simulink model "DesignTemperatureControlForDataCenter"  (R2025b)
settings: Solver=daessc  StartTime=0.0  StopTime=3600*4  FixedStep=0.5  MaxStep=1  RelTol=1e-3  AbsTol=1e-3
PreLoadFcn:
  | if ~exist("modelParam")
  |     setDefaultParameters;
  | end
undefined symbols (not defined in the file or in its folder): DiscIntNeverNeededParam, modelParam, value
libraries: fl_lib x78, nesl_utility x18, SimscapeFluids_lib x11, datacenter_lib x9, simulink_extras x4, slpidlib x2
(part 1 of 3)
settings Model: Creator=vikrants  LastModifiedBy=vikrants
settings SolverCC: AutoScaleAbsTol=off  NumberNewtonIterations=5.0  MaxConsecutiveMinStep=10  AlgebraicLoopSolver=TrustRegion  MaxZcPerStep=1.0
settings DataIOCC: SaveOutput=off  DSMLogging=off  SaveTime=off  ReturnWorkspaceOutputs=off  SignalLoggingName=logsout_DesignTemperatureControllerDataCenter
settings DebuggingCC: UnconnectedInputMsg=warning  UnconnectedOutputMsg=warning  UnconnectedLineMsg=warning  SymbolicDimsDataTypeCodeGenerationDiagnostic=none
settings ModelReferenceCC: EnableRefExpFcnMdlSchedulingChecks=on
settings SFSimCC: CustomCodeUndefinedFunction=UseInterfaceOnly
settings RTWCC: GPUComputeCapability=3.5  DLArmComputeVersion=19.05
settings SimscapeCC: SimscapeLogLimitData=off  SimscapeLogDataHistory=10000.0

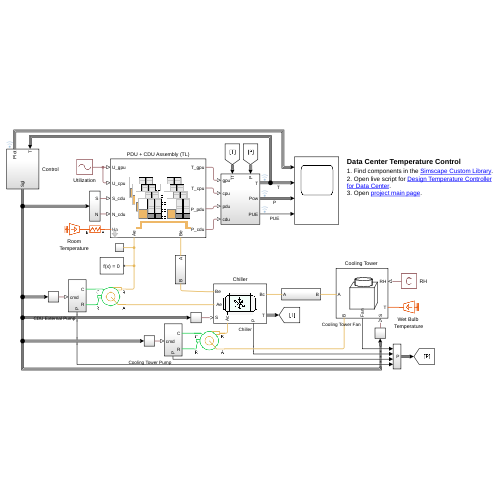
[thumbnail: Simulink's stored preview of the top-level diagram]
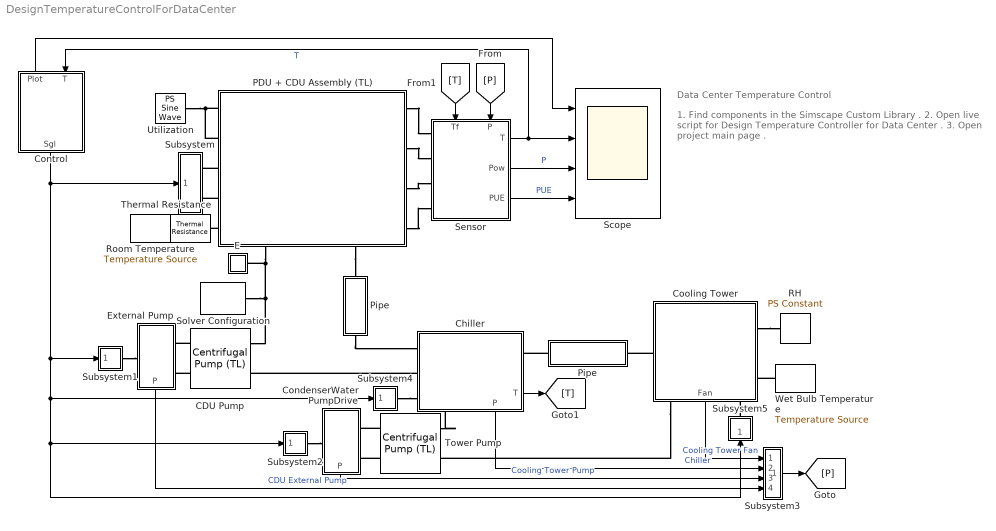
== system DesignTemperatureControlForDataCenter ==
  note: Data Center Temperature Control
  note: 1. Find components in the Simscape Custom Library .
      | 2. Open live script for Design Temperature Controller for Data Center .
      | 3. Open project main page .
  CDU Pump : SimscapeFluids_lib/Thermal Liquid/Pumps & Motors/Centrifugal Pump (TL)  pump_parameterization=fluids.thermal_liquid.pumps_motors.enum.CentrifugalPumpParameterization.Nominal  capacity_ref_nominal=5736% 07-Oct-2026 22:51:40 lpm  head_ref_nominal=33 m  power_ref_nominal=100 kW  head_ref_max=48 m  capacity_ref_max=16520% 07-Oct-2026 22:51:40 lpm  omega_ref_analytic=2400 rpm  flow_rate_1D_TLU=[16.67, 30, 40, 53.33, 66.67, 83.33] lpm  head_1D_TLU=[50, 47.5, 45, 40, 35, 25] m  power_1D_TLU=[.6, .75, .85, .93, .98, .99] kW  omega_ref_1D=3500 rpm  rho_ref_1D=998.21 kg/m^3  omega_threshold_factor=1e-2  flow_rate_2D_TLU=[16.67, 23.33, 30, 40, 53.33, 60] lpm  omega_2D_TLU=[2450, 2800, 3150, 3500] rpm  head_2D_TLU=[25, 32.7, 42.5, 50; 24, 31.7, 41, 49; 22.7, 30.5, 39, 47.5; 20, 28, 36, 45; 15.7, 24, 32, 40; 12.5, 21, 29.5, 37.5] m  power_2D_TLU=[.28, .38, .5, .6; .31, .41, .55, .68; .33, .44, .6, .75; .36, .48, .65, .83; .38, .53, .72, .93; .39, .55, .75, .97] kW  rho_ref_2D=998.21 kg/m^3  diameter_ratio=1  mech_orientation=fluids.thermal_liquid.pumps_motors.enum.CentrifugalPumpMechOrientation.Positive  area=0.01 m^2  operation_check=simscape.enum.assert.action.none
      settings: InternalSimscapePortConfiguration="{\"Bottom\":[],\"Left\":[{\"id\":\"A\",\"label\":\"A\",\"type\":\"foundation.thermal_liquid.thermal_liquid\"},{\"id\":\"B\",\"label\":\"B\",\"type\":\"foundation.thermal_liquid.thermal_liquid\"}],\"Right\":[{\"id\":\"R\",\"label\":\"R\",\"type\":\"foundation.mechanical.rotational.rotational\"},{\"id\":\"C\",\"label\":\"C\",\"type\":\"foundation.mechanical.rotational.rotational\"}],\"Top\":[]}"
  Chiller : Subsystem
      settings: PortSchema="{\"entries\":[{\"content\":{\"sides\":[{\"content\":{\"connectorIds\":[\"LConn1\",\"LConn2\",\"LConn3\"]},\"type\":\"ConnectorPlacement.EquallySpacedRectSide\",\"uuid\":\"5ed28ea1-4316-4f65-adaa-c4c395baecab\"},{\"content\":{\"connectorIds\":[\"RConn1\",\"Out1\"],\"side\":\"RIGHT\"},\"type\":\"ConnectorPlacement.EquallySpacedRectSide\",\"uuid\":\"be940e19-35ef-4c96-93bb-75051a224bd3\"},{\"content\":{\"side\":\"TOP\"},\"type\":\"ConnectorPlacement.EquallySpacedRectSide\",\"uuid\":\"b036d98d-44b0-4d36-b684-218fa73e271c\"},{\"content\":{\"connectorIds\":[\"RConn2\",\"Out2\"],\"side\":\"BOTTOM\"},\"type\":\"ConnectorPlacement.EquallySpacedRectSide\",\"uuid\":\"f31ac10c-e496-4b68-ab88-599a2fb40368\"}]},\"type\":\"ConnectorPlacement.EquallySpacedConnector\",\"uuid\":\"f19a8016-13fc-43c4-a484-59a5b5ad8f66\"}],\"packageUris\":[\"http://schema.mathworks.com/mf0/Connector/R2020b\"],\"version\":\"1.0\"}"
      mask Display: image('icon_Chiller.png');
  CondenserWater PumpDrive : Subsystem
      settings: PortSchema="{\"entries\":[{\"content\":{\"sides\":[{\"content\":{},\"type\":\"ConnectorPlacement.EquallySpacedRectSide\",\"uuid\":\"edaea338-c02b-45e4-bb82-2d3d355c0ecb\"},{\"content\":{\"connectorIds\":[\"Out1\"],\"side\":\"RIGHT\"},\"type\":\"ConnectorPlacement.EquallySpacedRectSide\",\"uuid\":\"dbf9c5c1-eafd-40d4-aa46-26e8ea9aa192\"},{\"content\":{\"connectorIds\":[\"LConn1\",\"LConn2\"],\"side\":\"TOP\"},\"type\":\"ConnectorPlacement.EquallySpacedRectSide\",\"uuid\":\"608efdba-9ff5-4da4-84d8-d12421fbb1b5\"},{\"content\":{\"connectorIds\":[\"RConn1\"],\"side\":\"BOTTOM\"},\"type\":\"ConnectorPlacement.EquallySpacedRectSide\",\"uuid\":\"608ab80a-f5e8-4836-b78e-f2f30ba8946b\"}]},\"type\":\"ConnectorPlacement.EquallySpacedConnector\",\"uuid\":\"d68ea5d9-0a41-4434-9ea5-6f17886b9eb3\"}],\"packageUris\":[\"http://schema.mathworks.com/mf0/Connector/R2020b\"],\"version\":\"1.0\"}"
  Control : Subsystem
      settings: PortSchema="{\"entries\":[{\"content\":{\"sides\":[{\"content\":{},\"type\":\"ConnectorPlacement.EquallySpacedRectSide\",\"uuid\":\"a63835dd-0736-4651-a3a6-af79242b31fb\"},{\"content\":{\"side\":\"RIGHT\"},\"type\":\"ConnectorPlacement.EquallySpacedRectSide\",\"uuid\":\"03a8bfb2-50d7-4ebf-813a-a0a6e11f28b8\"},{\"content\":{\"connectorIds\":[\"Out2\",\"In1\"],\"side\":\"TOP\"},\"type\":\"ConnectorPlacement.EquallySpacedRectSide\",\"uuid\":\"89fea5db-68ca-4c43-b344-545b60b759ce\"},{\"content\":{\"connectorIds\":[\"Out1\"],\"side\":\"BOTTOM\"},\"type\":\"ConnectorPlacement.EquallySpacedRectSide\",\"uuid\":\"0ca3921b-bf69-47aa-b890-d4c74b431990\"}]},\"type\":\"ConnectorPlacement.EquallySpacedConnector\",\"uuid\":\"7f07e0e8-2f26-4107-8e9d-e0237b0af823\"}],\"packageUris\":[\"http://schema.mathworks.com/mf0/Connector/R2020b\"],\"version\":\"1.0\"}"
  "Cooling Tower " : Subsystem
      settings: PortSchema="{\"entries\":[{\"content\":{\"sides\":[{\"content\":{\"connectorIds\":[\"LConn1\"]},\"type\":\"ConnectorPlacement.EquallySpacedRectSide\",\"uuid\":\"fb95f023-248b-4fd8-b2e8-d9442f9ed266\"},{\"content\":{\"connectorIds\":[\"RConn1\",\"RConn2\"],\"side\":\"RIGHT\"},\"type\":\"ConnectorPlacement.EquallySpacedRectSide\",\"uuid\":\"34018b48-7083-4d8d-9b59-330dd3458507\"},{\"content\":{\"side\":\"TOP\"},\"type\":\"ConnectorPlacement.EquallySpacedRectSide\",\"uuid\":\"5b7035e5-549d-4a54-bb0d-bc476d1d6775\"},{\"content\":{\"connectorIds\":[\"RConn3\",\"Out1\",\"RConn4\"],\"side\":\"BOTTOM\"},\"type\":\"ConnectorPlacement.EquallySpacedRectSide\",\"uuid\":\"6fdb7fbc-eae2-40f9-9e2f-d0242d275ed0\"}]},\"type\":\"ConnectorPlacement.EquallySpacedConnector\",\"uuid\":\"c33b1996-e402-4893-a457-f5cd841aa14c\"}],\"packageUris\":[\"http://schema.mathworks.com/mf0/Connector/R2020b\"],\"version\":\"1.0\"}"
      mask Display:
      | color('white')
      | plot(150, 150)
      | plot(-150, -180)
      | color('black')
      | 
      | % Number of points on arcs
      | n = 40;
      | 
      | y1 = 80;
      | w1 = 50;
      | h1 = 10;
      | 
      | y2 = 40;
      | y3 = -100;
      | w2 = 70;
      | h2 = 20;
      | 
      | % Cylinder
      | plot([-w1 -w1] + h2/2, [y1 y2])
      | plot([w1 w1] + h2/2, [y1 y2])
      | plot(cos(linspace(0, 2*pi, n))*w1 + h2/2, sin(linspace(0, 2*pi, n))*h1 + y1)
      | plot(cos(linspace(0, pi, n/2))*w1 + h2/2, -sin(linspace(0, pi, n/2))*h1 + y2)
      | 
      | % Box
      | plot([-w2 w2 w2 -w2 -w2], [y2 y2 y3 y3 y2]-h2)
      | plot([-w2+h2 -w1+h2/2], [y2+h2 y2+h2])
      | plot([w1+h2/2 w2+h2 w2+h2], [y2+h2 y2+h2 y3+h2])
      | plot([w2 w2+h2], [y2-h2 y2+h2])
      | plot([w2 w2+h2], [y3-h2 y3+h2])
      | plot([-w2 -w2+h2], [y2-h2 y2+h2])
  E : Subsystem
  External Pump : Subsystem
      settings: PortSchema="{\"entries\":[{\"content\":{\"sides\":[{\"content\":{},\"type\":\"ConnectorPlacement.EquallySpacedRectSide\",\"uuid\":\"edaea338-c02b-45e4-bb82-2d3d355c0ecb\"},{\"content\":{\"connectorIds\":[\"Out1\"],\"side\":\"RIGHT\"},\"type\":\"ConnectorPlacement.EquallySpacedRectSide\",\"uuid\":\"dbf9c5c1-eafd-40d4-aa46-26e8ea9aa192\"},{\"content\":{\"connectorIds\":[\"LConn1\",\"LConn2\"],\"side\":\"TOP\"},\"type\":\"ConnectorPlacement.EquallySpacedRectSide\",\"uuid\":\"608efdba-9ff5-4da4-84d8-d12421fbb1b5\"},{\"content\":{\"connectorIds\":[\"RConn1\"],\"side\":\"BOTTOM\"},\"type\":\"ConnectorPlacement.EquallySpacedRectSide\",\"uuid\":\"608ab80a-f5e8-4836-b78e-f2f30ba8946b\"}]},\"type\":\"ConnectorPlacement.EquallySpacedConnector\",\"uuid\":\"d68ea5d9-0a41-4434-9ea5-6f17886b9eb3\"}],\"packageUris\":[\"http://schema.mathworks.com/mf0/Connector/R2020b\"],\"version\":\"1.0\"}"
  PDU + CDU Assembly (TL) : Subsystem  mask{nAssembly=60, nTrays=6, nRacks=4, nPumps=2, pumpNominalRPM=3500, pumpCapacityVec=[0.1:0.1:1.2]/998, pumpRefHeadVec=[239, 238.5, 232, 230, 222, 216, 208, 196, 186, 170,150,130], pumpRefBrkPowVec=1000*[0.3,0.4,0.45,0.5,0.55,0.6,0.65,0.7,0.75,0.78,0.79,0.798], pumpEff=[20,40,50,60,65,70,75,75,75,73,68,60]/100, speedLimFactor=5, pumpImpellerDiaFactor=1, extFluidMdot=[.3, .5, 1, 1.3, 1.7, 2, 2.6, 3.3], extFluidPrDrop=0.1*[9,25,100,169,289,400,676,1090]%20*ones(1,8), extFluidVol=0.01, extFluidPipeArea=0.01*2, intFluidMdot=[.3, .5, .6, .7, 1, 1.4, 1.9, 2.3], intFluidPrDrop=[9,25,100,169,289,400,676,1090]*5%1000*ones(1,8), intFluidVol=0.01, intFluidPipeArea=0.01, spDissipationTbl=1000*[.324, .3533, .404, .4253, .4333, .4373, .4453, .4533; .3813, .424, .496, .5307, .544, .5547, .5693, .5787; .4267, .4827, .5813, .6173, .6413, .6573, .672, .6827; .4613, .528, .64, .6987, .7267, .7467, .7707, .7853; .5533, .6467, .8227, .928, .9853, 1.0187, 1.0653, 1.0973; .58, .688, .8853, 1.0147, 1.08, 1.124, 1.176, 1.2147; .624, .7467, .992, 1.148, 1.244, 1.304, 1.3773, 1.4267; .656, .7907, 1.0667, 1.26, 1.376, 1.452, 1.548, 1.612], effPipeLen=20, refT=293, refP=0.101325, refDensity=998, trayMass=15, trayCp=6000, trayThermalR=1e-3, nGPU=3, gpuTDPperDie=1200, gpuIdlePower=300, gpuHBMpower=80, gpuExponent=1.4, gpuHBMutil=0.7, gpuLeakage=1.5, gpuNominalDieT=350, gpuDieThermalC=50, gpuHeatSinkR=1e-3, gpuSurfArea=0.01, gpuAmbientR=1e-3, nCPU=1, cpuTDPperSocket=350, cpuIdlePower=80, cpuExponent=1.1, cpuLeakage=1.5, cpuNominalDieT=350, cpuDieThermalC=50, cpuHeatSinkR=1e-3, cpuSurfArea=0.01, cpuAmbientR=1e-3, initialT=max(274,value(modelParam.WetBulbT ,"K")), initialP=0.101325+0.01, htc=10}
      mask prompts: nAssembly "Number of PDU+CDU assemblies (-)"; nTrays "Number of IT trays per rack (-)"; nRacks "Number of racks (-)"; nPumps "Total number of pumps (-)"; pumpNominalRPM "Pump nominal rating (rpm)"; pumpCapacityVec "Reference capacity vector for each pump (m^3/s)"; pumpRefHeadVec "Reference head vector for each pump (m)"; pumpRefBrkPowVec "Reference brake power vector (kW)"; pumpEff "Electrical efficiency vector, 0-1 (-)"; speedLimFactor "Pump speed upper limit factor (-)"; pumpImpellerDiaFactor "Impeller diameter scale factor (-)"; extFluidMdot "External liquid loop mass flow rate vector (kg/s)"; extFluidPrDrop "External liquid loop pressure drop vector (kPa)"; extFluidVol "External liquid volume in heat exchanger (m^3)"; extFluidPipeArea "External liquid loop pipe cross-sectional area (m^2)"; intFluidMdot "Internal liquid loop mass flow rate vector (kg/s)"; intFluidPrDrop "Internal liquid loop pressure drop vector (kPa)"; intFluidVol "Internal liquid volume in heat exchanger (m^3)"; intFluidPipeArea "Internal liquid loop pipe cross-sectional area (m^2)"; spDissipationTbl "Specific dissipation table, SD[mdot_int,mdot_ext] (kW/K)"; effPipeLen "Effective pipe length for rack cooling (m)"; refT "Reference flow temperature (K)"; refP "Reference flow pressure (MPa)"; refDensity "Reference density for internal liquid (kg/m^3)"; trayMass "Tray mass (kg)"; trayCp "Tray specific heat capacity (J/kg*K)"; trayThermalR "Tray to external thermal resistance (K/W)"; nGPU "Number of GPU per tray (-)"; gpuTDPperDie "GPU TDP per die (W)"; gpuIdlePower "GPU idle power (W)"; gpuHBMpower "HBM power per GPU (W)"; gpuExponent "GPU power utilization exponent (-)"; gpuHBMutil "HBM utilization as fraction of compute utilization (-)"; gpuLeakage "Leakage increase per K above nominal temperature (W/K)"; gpuNominalDieT "Nominal die temperature at TDP (K)"; gpuDieThermalC "GPU die thermal capacitance (J/K)"; gpuHeatSinkR "GPU die-heat-sink thermal resistance (K/W)"; gpuSurfArea "Surface area per die for ambient heat transfer (m^2)"; gpuAmbientR "GPU die-ambient thermal resistance (K/W)"; nCPU "Number of CPU per tray (-)"; cpuTDPperSocket "CPU TDP per socket (W)"; cpuIdlePower "CPU idle power per socket (W)"; cpuExponent "CPU power utilization exponent (-)"; cpuLeakage "Leakage increase per K above nominal temperature (W/K)"; cpuNominalDieT "Nominal die temperature at TDP (K)"; cpuDieThermalC "CPU die thermal capacitance (J/K)"; cpuHeatSinkR "CPU die-heat-sink thermal resistance (K/W)"; cpuSurfArea "Surface area per die for ambient heat transfer (m^2)"; cpuAmbientR "CPU die-ambient thermal resistance (K/W)"; initialT "Initial temperature (K)"; initialP "Initial pressure (MPa)"; htc "Heat transfer coefficient to ambient (W/m^2.K)"
      settings: CopyFcn=set_param(gcbh,'LinkStatus','none');  PortSchema="{\"entries\":[{\"content\":{\"sides\":[{\"content\":{\"connectorIds\":[\"LConn1\",\"LConn2\",\"LConn3\",\"LConn4\",\"LConn5\"]},\"type\":\"ConnectorPlacement.EquallySpacedRectSide\",\"uuid\":\"c3c2deed-cbbd-4247-9ad8-92266cae4888\"},{\"content\":{\"connectorIds\":[\"RConn1\",\"RConn2\",\"RConn3\",\"RConn4\"],\"side\":\"RIGHT\"},\"type\":\"ConnectorPlacement.EquallySpacedRectSide\",\"uuid\":\"76c347ba-a09e-43ac-9cd7-77a64cbfa06b\"},{\"content\":{\"side\":\"TOP\"},\"type\":\"ConnectorPlacement.EquallySpacedRectSide\",\"uuid\":\"42a451f0-8c6e-4292-b7e5-775225f62bd3\"},{\"content\":{\"connectorIds\":[\"RConn5\",\"RConn6\"],\"side\":\"BOTTOM\"},\"type\":\"ConnectorPlacement.EquallySpacedRectSide\",\"uuid\":\"cd4c05de-d563-4aeb-b6ce-436a52495d26\"}]},\"type\":\"ConnectorPlacement.EquallySpacedConnector\",\"uuid\":\"03434805-a51b-483c-9948-e3fbab74b7d0\"}],\"packageUris\":[\"http://schema.mathworks.com/mf0/Connector/R2020b\"],\"version\":\"1.0\"}"
      mask Help: web("DocumentationPDUCDUAssemblyTL.html")
      mask DialogControl Container10 Prompt: PDU Racks
      mask DialogControl getRatingButton Prompt: Get Rating
      mask DialogControl Container5_2 Prompt: CDU
      mask DialogControl Container13 Prompt: Pumps
      mask DialogControl Container8_2 Prompt: Set External Fluid Properties
      mask DialogControl Container7_2 Prompt: Set Internal Fluid Properties
      mask DialogControl Container9_2 Prompt: Heat Transfer
      mask DialogControl Container14 Prompt: Reference Properties
      mask DialogControl Container9 Prompt: IT Tray
      mask DialogControl Container6 Prompt: GPU
      mask DialogControl Container7 Prompt: CPU
      mask DialogControl Container8 Prompt: Initial Conditions
      mask Display: image('icon_AssemblyTL.png');
  Pipe : Subsystem
  "Pipe " : Subsystem
  RH : fl_lib/Physical Signals/Sources/PS Constant  constant=modelParam.relHumidity
  Room Temperature : fl_lib/Thermal/Thermal Sources/Temperature Source  temperature="value(modelParam.RoomT,\"K\") K"
  Scope : Scope  NumInputPorts=4
      settings: ActiveDisplayYMinimum=-0.25  ActiveDisplayYMaximum=2.2500000000000004
  Sensor : Subsystem
      settings: PortSchema="{\"entries\":[{\"content\":{\"sides\":[{\"content\":{\"connectorIds\":[\"LConn1\",\"LConn2\",\"LConn3\",\"LConn4\"]},\"type\":\"ConnectorPlacement.EquallySpacedRectSide\",\"uuid\":\"6c5d1fe6-dd50-454a-84ba-53430ab87bc5\"},{\"content\":{\"connectorIds\":[\"Out1\",\"Out2\",\"Out3\"],\"side\":\"RIGHT\"},\"type\":\"ConnectorPlacement.EquallySpacedRectSide\",\"uuid\":\"d5157b7a-8f4f-4e82-afe2-1817efbe5600\"},{\"content\":{\"connectorIds\":[\"In1\",\"In2\"],\"side\":\"TOP\"},\"type\":\"ConnectorPlacement.EquallySpacedRectSide\",\"uuid\":\"009318cb-beda-4b27-8dc1-f51e5342655e\"},{\"content\":{\"side\":\"BOTTOM\"},\"type\":\"ConnectorPlacement.EquallySpacedRectSide\",\"uuid\":\"86d00183-87c9-4506-a12a-6ddd83a55427\"}]},\"type\":\"ConnectorPlacement.EquallySpacedConnector\",\"uuid\":\"e26bc32b-3d15-4893-9174-56352d5e9e55\"}],\"packageUris\":[\"http://schema.mathworks.com/mf0/Connector/R2020b\"],\"version\":\"1.0\"}"
  Solver Configuration : nesl_utility/Solver Configuration  PhysicalDomain=network_engine_domain  SubClassName=solver  LeftPortType=input  RightPortType=generic  Tones=[]  Harmonics=[]  SimulateNoise=off  Profile=off  UseLocalSampling=off  EnableSwitchedLinearOptims=on  FrequencyDomain=off  UseCCode=off  RelTol=0.001  AbsTol=1e-06  MinStep=1e-09  ToWorkspace=off  RevertToSquareIcSolve=off  NumHomotopyIterations=100  PhasorMode=off  PhasorModeNumHarmonics=1  ConsistencySolver=NEWTON_XTOL_AFTER_FTOL  IndexReductionMethod=DerivativeReplacement  DoDC=off  ResidualTolerance=1e-09  ConsistencyTolSource=GLOBAL  ConsistencyAbsTol=0.001  ConsistencyRelTol=0.001  ConsistencyTolFactor=0.001  UseLocalSolver=off  LocalSolverChoice=NE_BACKWARD_EULER_ADVANCER  ResolveIndetEquations=on  FunctionEvalNumThread=1  LocalSolverSampleTime=0.001  DoFixedCost=off  MaxNonlinIter=3  MaxModeIter=2  ComputeImpulses=off  ImpulseIterations=2  LinearAlgebra=auto  LinearAlgebraNumThread=0  EquationFormulation=NE_TIME_EF  DelaysMemoryBudget=1024  AutomaticFiltering=on  FilteringTimeConstant=0.001  PartitionStorageMethod=AS_NEEDED  PartitionMemoryBudget=1024  PartitionMethod=ROBUST  MultibodyUseLocalSolver=off  MultibodyLocalSolverChoice=ODE1  MultibodyLocalSolverSampleTime=0.001
  Subsystem : Subsystem
  Subsystem1 : Subsystem
  Subsystem2 : Subsystem
  Subsystem3 : Subsystem
  Subsystem4 : Subsystem
  Subsystem5 : Subsystem
  Thermal Resistance : fl_lib/Thermal/Thermal Elements/Thermal Resistance  resistance=1e-2 K/W  T_specify=off  T_priority=None  T=0 K  T_nominal_specify=off  T_nominal_value=1  T_nominal_unit=K  Q_specify=off  Q_priority=None  Q=0 W  Q_nominal_specify=off  Q_nominal_value=1  Q_nominal_unit=W
  Tower Pump : SimscapeFluids_lib/Thermal Liquid/Pumps & Motors/Centrifugal Pump (TL)  pump_parameterization=fluids.thermal_liquid.pumps_motors.enum.CentrifugalPumpParameterization.Nominal  capacity_ref_nominal=5736% 07-Oct-2026 22:51:40 lpm  head_ref_nominal=33 m  power_ref_nominal=100 kW  head_ref_max=48 m  capacity_ref_max=16520% 07-Oct-2026 22:51:40 lpm  omega_ref_analytic=2400 rpm  flow_rate_1D_TLU=[16.67, 30, 40, 53.33, 66.67, 83.33] lpm  head_1D_TLU=[50, 47.5, 45, 40, 35, 25] m  power_1D_TLU=[.6, .75, .85, .93, .98, .99] kW  omega_ref_1D=3500 rpm  rho_ref_1D=998.21 kg/m^3  omega_threshold_factor=1e-2  flow_rate_2D_TLU=[16.67, 23.33, 30, 40, 53.33, 60] lpm  omega_2D_TLU=[2450, 2800, 3150, 3500] rpm  head_2D_TLU=[25, 32.7, 42.5, 50; 24, 31.7, 41, 49; 22.7, 30.5, 39, 47.5; 20, 28, 36, 45; 15.7, 24, 32, 40; 12.5, 21, 29.5, 37.5] m  power_2D_TLU=[.28, .38, .5, .6; .31, .41, .55, .68; .33, .44, .6, .75; .36, .48, .65, .83; .38, .53, .72, .93; .39, .55, .75, .97] kW  rho_ref_2D=998.21 kg/m^3  diameter_ratio=1  mech_orientation=fluids.thermal_liquid.pumps_motors.enum.CentrifugalPumpMechOrientation.Positive  area=0.01 m^2  operation_check=simscape.enum.assert.action.none
      settings: InternalSimscapePortConfiguration="{\"Bottom\":[],\"Left\":[{\"id\":\"A\",\"label\":\"A\",\"type\":\"foundation.thermal_liquid.thermal_liquid\"},{\"id\":\"B\",\"label\":\"B\",\"type\":\"foundation.thermal_liquid.thermal_liquid\"}],\"Right\":[{\"id\":\"R\",\"label\":\"R\",\"type\":\"foundation.mechanical.rotational.rotational\"},{\"id\":\"C\",\"label\":\"C\",\"type\":\"foundation.mechanical.rotational.rotational\"}],\"Top\":[]}"
  Utilization : fl_lib/Physical Signals/Sources/PS Sine Wave  amplitude=0.49  bias=0.5  frequency_spec=foundation.enum.frequencySpec.frequencySI  frequency_SI=1/(600) Hz  frequency_angular=1 rad/s  phase=0 rad
      settings: InternalSimscapePortConfiguration="{\"Bottom\":[],\"Left\":[],\"Right\":[{\"id\":\"O\",\"label\":\"\",\"type\":\"output\"}],\"Top\":[]}"
  Wet Bulb Temperature : fl_lib/Thermal/Thermal Sources/Temperature Source  temperature="value(modelParam.WetBulbT ,\"K\") K"
  wires:
  Subsystem3/1(P) -> [P]
  Chiller/1(T) -> [T]
  Sensor/1(T) -> Scope/2, Control/1(T)  "T"
  [T] -> Sensor/1(Tf)
  [P] -> Sensor/2(P)
  Sensor/2(Pow) -> Scope/3  "P"
  Sensor/3(PUE) -> Scope/4  "PUE"
  Control/1(Sgl) -> Subsystem5/1(" "), Subsystem2/1(" "), Subsystem4/1(" "), Subsystem1/1(" "), Subsystem/1(" ")
  Control/2(Plot) -> Scope/1
  "Cooling Tower "/1(Fan) -> Subsystem3/1("    ")  "Cooling Tower Fan"
  Chiller/2(P) -> Subsystem3/2("   ")  "Chiller"
  CondenserWater PumpDrive/1(P) -> Subsystem3/3("  ")  "Cooling Tower Pump"
  External Pump/1(P) -> Subsystem3/4(" ")  "CDU External Pump"
  connections:
  PDU + CDU Assembly (TL)/LConn5 -- Thermal Resistance/LConn1
  Room Temperature/LConn1 -- Thermal Resistance/RConn1
  Tower Pump/RConn2 -- CondenserWater PumpDrive/LConn1
  Tower Pump/RConn1 -- CondenserWater PumpDrive/LConn2
  Utilization/RConn1 -- PDU + CDU Assembly (TL)/LConn2 -- PDU + CDU Assembly (TL)/LConn1
  CDU Pump/LConn2 -- Solver Configuration/RConn1 -- PDU + CDU Assembly (TL)/RConn5 -- E/LConn1
  CDU Pump/RConn1 -- External Pump/LConn2
  CDU Pump/RConn2 -- External Pump/LConn1
  PDU + CDU Assembly (TL)/RConn6 -- Pipe/LConn1
  "Cooling Tower "/LConn1 -- "Pipe "/RConn1
  "Cooling Tower "/RConn3 -- Tower Pump/LConn1
  "Cooling Tower "/RConn1 -- RH/RConn1
  Wet Bulb Temperature/LConn1 -- "Cooling Tower "/RConn2
  "Pipe "/LConn1 -- Chiller/RConn1
  Tower Pump/LConn2 -- Chiller/RConn2
  PDU + CDU Assembly (TL)/RConn1 -- Sensor/LConn1
  PDU + CDU Assembly (TL)/RConn2 -- Sensor/LConn2
  PDU + CDU Assembly (TL)/RConn3 -- Sensor/LConn3
  PDU + CDU Assembly (TL)/RConn4 -- Sensor/LConn4
  Pipe/RConn1 -- Chiller/LConn1
  Chiller/LConn2 -- CDU Pump/LConn1
  PDU + CDU Assembly (TL)/LConn3 -- Subsystem/RConn1
  PDU + CDU Assembly (TL)/LConn4 -- Subsystem/RConn2
  Subsystem1/RConn1 -- External Pump/RConn1
  Subsystem2/RConn1 -- CondenserWater PumpDrive/RConn1
  Subsystem4/RConn1 -- Chiller/LConn3
  Subsystem5/RConn1 -- "Cooling Tower "/RConn4

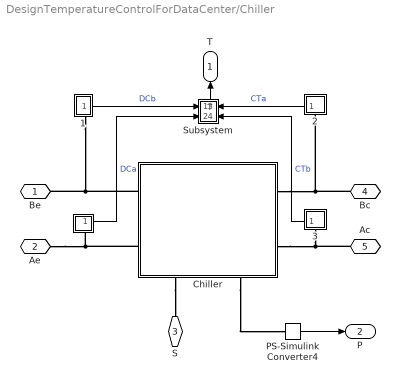
== system DesignTemperatureControlForDataCenter/Chiller ==
  "   " : Subsystem
      settings: PortSchema="{\"entries\":[{\"content\":{\"sides\":[{\"content\":{\"connectorIds\":[\"Out1\"]},\"type\":\"ConnectorPlacement.EquallySpacedRectSide\",\"uuid\":\"3399dc99-4627-40d0-8367-e96dc72dde0c\"},{\"content\":{\"side\":\"RIGHT\"},\"type\":\"ConnectorPlacement.EquallySpacedRectSide\",\"uuid\":\"2ba4a119-1ff0-405b-91c6-ea11b86558ba\"},{\"content\":{\"side\":\"TOP\"},\"type\":\"ConnectorPlacement.EquallySpacedRectSide\",\"uuid\":\"f574a1ad-8559-46c9-b8f5-c615fa71de09\"},{\"content\":{\"connectorIds\":[\"RConn1\"],\"side\":\"BOTTOM\"},\"type\":\"ConnectorPlacement.EquallySpacedRectSide\",\"uuid\":\"c607c849-0183-47f5-8d51-60dde6823f3f\"}]},\"type\":\"ConnectorPlacement.EquallySpacedConnector\",\"uuid\":\"8117aef0-2106-4d3a-b9fb-cd5d36b9a7b7\"}],\"packageUris\":[\"http://schema.mathworks.com/mf0/Connector/R2020b\"],\"version\":\"1.0\"}"
  "   1" : Subsystem
      settings: PortSchema="{\"entries\":[{\"content\":{\"sides\":[{\"content\":{},\"type\":\"ConnectorPlacement.EquallySpacedRectSide\",\"uuid\":\"3399dc99-4627-40d0-8367-e96dc72dde0c\"},{\"content\":{\"connectorIds\":[\"RConn1\"],\"side\":\"RIGHT\"},\"type\":\"ConnectorPlacement.EquallySpacedRectSide\",\"uuid\":\"2ba4a119-1ff0-405b-91c6-ea11b86558ba\"},{\"content\":{\"side\":\"TOP\"},\"type\":\"ConnectorPlacement.EquallySpacedRectSide\",\"uuid\":\"f574a1ad-8559-46c9-b8f5-c615fa71de09\"},{\"content\":{\"connectorIds\":[\"Out1\"],\"side\":\"BOTTOM\"},\"type\":\"ConnectorPlacement.EquallySpacedRectSide\",\"uuid\":\"5a97e7e4-0942-4884-adac-89deb46a13da\"}]},\"type\":\"ConnectorPlacement.EquallySpacedConnector\",\"uuid\":\"8117aef0-2106-4d3a-b9fb-cd5d36b9a7b7\"}],\"packageUris\":[\"http://schema.mathworks.com/mf0/Connector/R2020b\"],\"version\":\"1.0\"}"
  "   2" : Subsystem
      settings: PortSchema="{\"entries\":[{\"content\":{\"sides\":[{\"content\":{},\"type\":\"ConnectorPlacement.EquallySpacedRectSide\",\"uuid\":\"3399dc99-4627-40d0-8367-e96dc72dde0c\"},{\"content\":{\"connectorIds\":[\"RConn1\"],\"side\":\"RIGHT\"},\"type\":\"ConnectorPlacement.EquallySpacedRectSide\",\"uuid\":\"2ba4a119-1ff0-405b-91c6-ea11b86558ba\"},{\"content\":{\"connectorIds\":[\"Out1\"],\"side\":\"TOP\"},\"type\":\"ConnectorPlacement.EquallySpacedRectSide\",\"uuid\":\"f574a1ad-8559-46c9-b8f5-c615fa71de09\"},{\"content\":{\"side\":\"BOTTOM\"},\"type\":\"ConnectorPlacement.EquallySpacedRectSide\",\"uuid\":\"b4b64539-20fe-4720-8e7b-f4bb537d6ab4\"}]},\"type\":\"ConnectorPlacement.EquallySpacedConnector\",\"uuid\":\"8117aef0-2106-4d3a-b9fb-cd5d36b9a7b7\"}],\"packageUris\":[\"http://schema.mathworks.com/mf0/Connector/R2020b\"],\"version\":\"1.0\"}"
  "   3" : Subsystem
      settings: PortSchema="{\"entries\":[{\"content\":{\"sides\":[{\"content\":{\"connectorIds\":[\"LConn1\"]},\"type\":\"ConnectorPlacement.EquallySpacedRectSide\",\"uuid\":\"3399dc99-4627-40d0-8367-e96dc72dde0c\"},{\"content\":{\"side\":\"RIGHT\"},\"type\":\"ConnectorPlacement.EquallySpacedRectSide\",\"uuid\":\"2ba4a119-1ff0-405b-91c6-ea11b86558ba\"},{\"content\":{\"connectorIds\":[\"Out1\"],\"side\":\"TOP\"},\"type\":\"ConnectorPlacement.EquallySpacedRectSide\",\"uuid\":\"f574a1ad-8559-46c9-b8f5-c615fa71de09\"},{\"content\":{\"side\":\"BOTTOM\"},\"type\":\"ConnectorPlacement.EquallySpacedRectSide\",\"uuid\":\"5977e3f4-33ad-4118-8448-d427b3e92e69\"}]},\"type\":\"ConnectorPlacement.EquallySpacedConnector\",\"uuid\":\"8117aef0-2106-4d3a-b9fb-cd5d36b9a7b7\"}],\"packageUris\":[\"http://schema.mathworks.com/mf0/Connector/R2020b\"],\"version\":\"1.0\"}"
  Chiller : Subsystem  mask{nominalRating=1500, nominalFlowrate=2*str2double(get_param("DesignTemperatureControlForDataCenter/PDU + CDU Assembly (TL)","nAssembly")), nominalPrDrop=1e-3, cop=9, volume=5, portArea=0.01, initialP=0.101325, initialT=max(274,value(modelParam.WetBulbT ,"K"))}
      mask prompts: nominalRating "Nominal rating (kW)"; nominalFlowrate "Nominal flowrate (kg/s)"; nominalPrDrop "Nominal pressure drop (MPa)"; cop "Coefficient of performance (-)"; volume "Chiller volume (m^3)"; portArea "Cross-sectional port area (m^2)"; initialP "Initial pressure (MPa)"; initialT "Initial temperature (K)"
      settings: CopyFcn=set_param(gcbh,'LinkStatus','none');  PortSchema="{\"entries\":[{\"content\":{\"sides\":[{\"content\":{\"connectorIds\":[\"LConn1\",\"LConn2\"]},\"type\":\"ConnectorPlacement.EquallySpacedRectSide\",\"uuid\":\"7d4232d9-e275-4255-9dc4-bc3f1c69ec46\"},{\"content\":{\"connectorIds\":[\"RConn1\",\"RConn2\"],\"side\":\"RIGHT\"},\"type\":\"ConnectorPlacement.EquallySpacedRectSide\",\"uuid\":\"7ca0ea83-7974-4453-97b6-22bfcf77b4f1\"},{\"content\":{\"connectorIds\":[\"LConn3\",\"LConn4\"],\"side\":\"TOP\"},\"type\":\"ConnectorPlacement.EquallySpacedRectSide\",\"uuid\":\"65c43657-b3f1-43d9-9625-8376acff2e22\"},{\"content\":{\"side\":\"BOTTOM\"},\"type\":\"ConnectorPlacement.EquallySpacedRectSide\",\"uuid\":\"1eb88563-12e2-4927-be7c-afaa658f242e\"}]},\"type\":\"ConnectorPlacement.EquallySpacedConnector\",\"uuid\":\"9af448fb-8903-42ba-af4c-44d5135333f1\"}],\"packageUris\":[\"http://schema.mathworks.com/mf0/Connector/R2020b\"],\"version\":\"1.0\"}"
      mask Help: web('DocumentationChiller.html')
      mask DialogControl Container2 Prompt: Rating
      mask DialogControl Container3 Prompt: Initial Conditions
      mask Display: image('icon_Chiller.png');
  PS-Simulink Converter4 : nesl_utility/PS-Simulink Converter  PhysicalDomain=network_engine_domain  SubClassName=ps_output  LeftPortType=input  RightPortType=output  PseudoPeriodic=off  Frequencies=[]  VectorFormat=inherit  Unit=inherit  AffineConversion=off
  Subsystem : Subsystem
      settings: PortSchema="{\"entries\":[{\"content\":{\"sides\":[{\"content\":{\"connectorIds\":[\"In1\",\"In2\"]},\"type\":\"ConnectorPlacement.EquallySpacedRectSide\",\"uuid\":\"da8d1222-07f1-4b52-a461-a0063c599c09\"},{\"content\":{\"connectorIds\":[\"In3\",\"In4\"],\"side\":\"RIGHT\"},\"type\":\"ConnectorPlacement.EquallySpacedRectSide\",\"uuid\":\"9a084b9a-e974-43b2-be24-72450e85e092\"},{\"content\":{\"connectorIds\":[\"Out1\"],\"side\":\"TOP\"},\"type\":\"ConnectorPlacement.EquallySpacedRectSide\",\"uuid\":\"604108f3-a25d-47a5-a80e-f070253abbf1\"}]},\"type\":\"ConnectorPlacement.EquallySpacedConnector\",\"uuid\":\"4a98f8aa-6861-4a99-b04b-9754ba5db579\"}],\"packageUris\":[\"http://schema.mathworks.com/mf0/Connector/R2020b\"],\"version\":\"1.0\"}"
  Be : PMIOPort  Side=Left
  " Ae" : PMIOPort  Port=2  Side=Left
  S : PMIOPort  Port=3  Side=Left
  Bc : PMIOPort  Port=4  Side=Right
  " Ac" : PMIOPort  Port=5  Side=Right
  T : Outport
  P : Outport  Port=2
  wires:
  "   3"/1(T) -> Subsystem/4("  ")  "CTb"
  "   1"/1(T) -> Subsystem/1("    ")  "DCb"
  "   "/1(T) -> Subsystem/2("   ")  "DCa"
  Subsystem/1(T) -> T/1
  "   2"/1(T) -> Subsystem/3(" ")  "CTa"
  PS-Simulink Converter4/1 -> P/1
  connections:
  "   3"/LConn1 -- Chiller/RConn1 -- " Ac"/RConn1
  Bc/RConn1 -- Chiller/RConn2 -- "   2"/RConn1
  " Ae"/RConn1 -- Chiller/LConn1 -- "   "/RConn1
  "   1"/RConn1 -- Chiller/LConn2 -- Be/RConn1
  Chiller/LConn3 -- S/RConn1
  Chiller/LConn4 -- PS-Simulink Converter4/LConn1

== system DesignTemperatureControlForDataCenter/CondenserWater PumpDrive ==
  Ideal Angular Velocity Source : fl_lib/Mechanical/Mechanical Sources/Ideal Angular Velocity Source
  Ideal Torque Sensor : fl_lib/Mechanical/Mechanical Sensors/Ideal Torque Sensor
  Mechanical Rotational Reference : fl_lib/Mechanical/Rotational Elements/Mechanical Rotational Reference
  PS Product : fl_lib/Physical Signals/Functions/PS Product
  PS-Simulink Converter3 : nesl_utility/PS-Simulink Converter  PhysicalDomain=network_engine_domain  SubClassName=ps_output  LeftPortType=input  RightPortType=output  PseudoPeriodic=off  Frequencies=[]  VectorFormat=inherit  Unit=inherit  AffineConversion=off
  Pump Speed : fl_lib/Physical Signals/Functions/PS Gain  gain=2400 rpm
  C : PMIOPort  Side=Left
  R : PMIOPort  Port=2  Side=Left
  cmd : PMIOPort  Port=3  Side=Right
  P : Outport
  wires:
  PS-Simulink Converter3/1 -> P/1  "P"
  connections:
  C/RConn1 -- Ideal Angular Velocity Source/RConn2 -- Mechanical Rotational Reference/LConn1
  Pump Speed/RConn1 -- PS Product/LConn2 -- Ideal Angular Velocity Source/RConn1
  cmd/RConn1 -- Pump Speed/LConn1
  Ideal Angular Velocity Source/LConn1 -- Ideal Torque Sensor/LConn1
  Ideal Torque Sensor/RConn1 -- R/RConn1
  Ideal Torque Sensor/RConn2 -- PS Product/LConn1
  PS-Simulink Converter3/LConn1 -- PS Product/RConn1

== system DesignTemperatureControlForDataCenter/Control ==
  T : Inport
  Bus Creator1 : BusCreator  Inputs=3
  Bus Creator2 : BusCreator  Inputs=2
  CDU Control : Subsystem  mask{deltaK=modelParam.NoPumpWindowT, nPumps=2, motorSpeed=0.01, pidP=100, pidI=10, pidD=1, delaySec=1}
      mask prompts: deltaK "Temperature window for no pumping (K)"; nPumps "Number of CDU pumps (-)"; motorSpeed "Minimum speed ratio of pump motor, 0-1 (-)"; pidP "PID controller P value"; pidI "PID controller I value"; pidD "PID controller D value"; delaySec "Measurement delay (s)"
      mask DialogControl Container2 Prompt: Measurements
      mask DialogControl Container3 Prompt: Control
  Chiller and Pump Control : Subsystem  mask{degC=value(modelParam.WaterSupplyTempCDU,"degC"), controllerP=0.1, controllerI=0.001, deltaT=modelParam.StepControlTempr, delaySec=1}
      mask prompts: degC "Cold water temperature to CDU (deg C)"; controllerP "PI controller P value (-)"; controllerI "PI controller I value (-)"; deltaT "Discrete temperature step control (deg C)"; delaySec "Measurement delay (s)"
      mask DialogControl Container2 Prompt: Chiller
      mask DialogControl Container3 Prompt: Condenser Pump
  Data : BusSelector  OutputSignals=DCa,DCb,CTa,CTb,Chip
  Subsystem1 : Subsystem
  Tset : Constant  Value=300
  Sgl : Outport
  Plot : Outport  Port=2
  wires:
  Bus Creator2/1 -> Plot/1, Sgl/1  "S"
  T/1 -> Data/1
  Data/5 -> CDU Control/1("Tc ")  "<Chip>"
  Bus Creator1/1 -> Bus Creator2/1  "Facilities"
  CDU Control/1(C) -> Subsystem1/1(S), Bus Creator2/2  "CDU"
  Tset/1 -> CDU Control/2("Ts ")
  Data/1 -> Chiller and Pump Control/1(<DCa>)  "<DCa>"
  Data/2 -> Chiller and Pump Control/2(<DCb>)  "<DCb>"
  Data/3 -> Chiller and Pump Control/3(<CTa>)  "<CTa>"
  Data/4 -> Chiller and Pump Control/4(<CTb>)  "<CTb>"
  Chiller and Pump Control/2(Chiller) -> Bus Creator1/2  "Chiller"
  Chiller and Pump Control/1(St) -> Bus Creator1/1  "Tower pump"
  Subsystem1/1(P) -> Bus Creator1/3  "CDU External Pump"

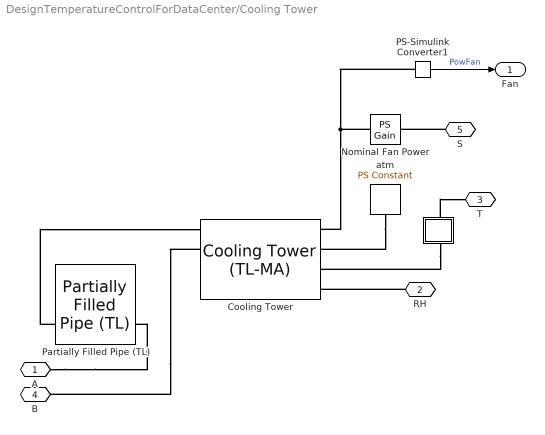
== system DesignTemperatureControlForDataCenter/Cooling Tower  ==
  " " : Subsystem
      settings: PortSchema="{\"entries\":[{\"content\":{\"sides\":[{\"content\":{},\"type\":\"ConnectorPlacement.EquallySpacedRectSide\",\"uuid\":\"58ecae8a-ee38-429b-b950-547b953091ad\"},{\"content\":{\"side\":\"RIGHT\"},\"type\":\"ConnectorPlacement.EquallySpacedRectSide\",\"uuid\":\"5811a52b-5b20-4d1a-9c02-75b130426e23\"},{\"content\":{\"connectorIds\":[\"LConn1\"],\"side\":\"TOP\"},\"type\":\"ConnectorPlacement.EquallySpacedRectSide\",\"uuid\":\"87b77f0f-9a0e-49e7-94ff-12e7a4b48565\"},{\"content\":{\"connectorIds\":[\"RConn1\"],\"side\":\"BOTTOM\"},\"type\":\"ConnectorPlacement.EquallySpacedRectSide\",\"uuid\":\"66a2e181-ef4b-4080-91ff-570337731427\"}]},\"type\":\"ConnectorPlacement.EquallySpacedConnector\",\"uuid\":\"2a8ea285-f75b-47f9-a527-b86403f3276b\"}],\"packageUris\":[\"http://schema.mathworks.com/mf0/Connector/R2020b\"],\"version\":\"1.0\"}"
      mask Display: disp('T');
  Cooling Tower : SimscapeFluids_lib/Heat Exchangers/Thermal Liquid - Moist Air/Cooling Tower (TL-MA)  flow_arrangement=fluids.heat_exchangers.enum.CoolingTowerFlowArrangement.Counter  capacity_spec_nominal_TL=fluids.heat_exchangers.enum.CoolingTowerCapacitySpecTL.VolumetricFlow  mdot_nominal_TL=42.7 kg/s  q_nominal_TL=modelParam.CoolingTower.Capacity lpm  Q_tower_nominal=1000 kW  Q_evap_nominal=800 kW  T_in_nominal_TL=28 degC  T_out_nominal_TL=22 degC  basin_model_TL=true  basin_area_TL=0.01*10 m^2  area_A1=0.01*10 m^2  area_B1=0.01*10 m^2  drift_rate_TL=0  auto_replenish_TL=true  T_makeup_TL=20 degC  nominal_init_TL=true  T_init_TL=29.44 degC  level_init_TL=0.5 m  g_TL=9.81 m/s^2  operating_conditions_MA=fluids.heat_exchangers.enum.CoolingTowerOperatingConditionsMA.InputSignals  flow_rate_spec_MA=fluids.heat_exchangers.enum.CoolingTowerFlowRateSpecMA.FanPower  output_power_MA=false  power_nominal_MA=45 kW  humidity_spec_MA=foundation.enum.HumiditySpec.RelativeHumidity  input_error_spec_MA=foundation.enum.input_range_error.warn  full_nominal_condition_MA=true  flow_rate_spec_nominal_MA=foundation.enum.mass_volumetric_flow.volumetric  mdot_nominal_MA=36 kg/s  q_nominal_MA=218 m^3/s  delta_p_nominal_MA=250 Pa  p_in_nominal_MA=0.101325 MPa  T_in_nominal_MA=20 degC  humidity_spec_nominal_MA=foundation.enum.HumiditySpec.RelativeHumidity  RH_in_nominal_MA=0.6  x_w_in_nominal_MA=0.0167  y_w_in_nominal_MA=0.0266  HR_in_nominal_MA=0.017  Tw_in_nominal_MA=25.56 degC  trace_gas_spec_nominal_MA=foundation.enum.trace_gas_spec.mass_fraction  x_g_in_nominal_MA=6e-4  y_g_in_nominal_MA=4e-4  volume_MA=24 m^3  area_A2=4 m^2  area_B2=4 m^2  nominal_init_MA=true  p_init_MA=0.101325 MPa  T_init_MA=34.28 degC  humidity_spec_init_MA=foundation.enum.HumiditySpec.WetBulbTemperature  RH_init_MA=0.5  x_w_init_MA=0.0167  y_w_init_MA=0.0266  HR_init_MA=0.017  Tw_init_MA=25.56 degC  trace_gas_spec_init_MA=foundation.enum.trace_gas_spec.mass_fraction  x_g_init_MA=6e-4  y_g_init_MA=4e-4  r_d_init_MA=0  RH_ws_MA=1  time_constant_cond_MA=1e-3 s  time_constant_evap_MA=1e-3 s  fraction_entrained_MA=1
      settings: InternalSimscapePortConfiguration="{\"Bottom\":[],\"Left\":[{\"id\":\"A1\",\"label\":\"A1\",\"type\":\"foundation.thermal_liquid.thermal_liquid\"},{\"id\":\"B1\",\"label\":\"B1\",\"type\":\"foundation.thermal_liquid.thermal_liquid\"}],\"Right\":[{\"id\":\"Pwr_in\",\"label\":\"Pwr\",\"type\":\"input\"},{\"id\":\"P\",\"label\":\"P\",\"type\":\"input\"},{\"id\":\"T\",\"label\":\"T\",\"type\":\"input\"},{\"id\":\"W\",\"label\":\"W\",\"type\":\"input\"}],\"Top\":[{\"id\":\"Q\",\"label\":\"Q\",\"type\":\"output\"},{\"id\":\"E\",\"label\":\"E\",\"type\":\"output\"}]}"
  Nominal Fan Power : fl_lib/Physical Signals/Functions/PS Gain  gain=45000 W
  PS-Simulink Converter1 : nesl_utility/PS-Simulink Converter  PhysicalDomain=network_engine_domain  SubClassName=ps_output  LeftPortType=input  RightPortType=output  PseudoPeriodic=off  Frequencies=[]  VectorFormat=inherit  Unit=inherit  AffineConversion=off
  Partially Filled Pipe (TL) : SimscapeFluids_lib/Thermal Liquid/Pipes & Fittings/Partially Filled Pipe (TL)  length=1 m  area=0.01*10 m^2  Dh=sqrt(4*0.01/pi) m  elevation_drop=1 m  level_init=1 m  level_check=simscape.enum.assert.action.error  g=9.81 m/s^2  length_add=1 m  roughness=15e-6 m  Re_lam=2000  Re_tur=4000  shape_factor=64  T0=28 degC
      settings: InternalSimscapePortConfiguration="{\"Bottom\":[{\"id\":\"B\",\"label\":\"B\",\"type\":\"foundation.thermal_liquid.thermal_liquid\"}],\"Left\":[{\"id\":\"AL\",\"label\":\"AL\",\"type\":\"input\"}],\"Right\":[{\"id\":\"L\",\"label\":\"L\",\"type\":\"output\"}],\"Top\":[{\"id\":\"A\",\"label\":\"A\",\"type\":\"foundation.thermal_liquid.thermal_liquid\"}]}"
  atm : fl_lib/Physical Signals/Sources/PS Constant  constant=1 atm
  A : PMIOPort  Side=Left
  RH : PMIOPort  Port=2  Side=Right
  T : PMIOPort  Port=3  Side=Right
  B : PMIOPort  Port=4  Side=Right
  S : PMIOPort  Port=5  Side=Right
  Fan : Outport
  wires:
  PS-Simulink Converter1/1 -> Fan/1  "PowFan"
  connections:
  PS-Simulink Converter1/LConn1 -- Cooling Tower/RConn1 -- Nominal Fan Power/RConn1
  Partially Filled Pipe (TL)/LConn2 -- Cooling Tower/LConn1
  S/RConn1 -- Nominal Fan Power/LConn1
  Cooling Tower/LConn2 -- B/RConn1
  A/RConn1 -- Partially Filled Pipe (TL)/RConn2
  RH/RConn1 -- Cooling Tower/RConn4
  atm/RConn1 -- Cooling Tower/RConn2
  " "/LConn1 -- T/RConn1
  " "/RConn1 -- Cooling Tower/RConn3

== system DesignTemperatureControlForDataCenter/E ==
  Expansion Tank : SimscapeFluids_lib/Thermal Liquid/Tanks & Accumulators/Gas-Charged Accumulator (TL)  capacity=1 m^3  dead_volume=1e-3 m^3  p_precharge_gauge=0.101313 MPa  k_sh=1.4  area=0.01 m^2  stiff_coeff=1e4 MPa/m^3  damping_coeff=1e4 MPa*s/m^6  liquid_volume_specify=on  liquid_volume_priority=None  liquid_volume=0.05 m^3  liquid_volume_nominal_specify=off  liquid_volume_nominal_value=1  liquid_volume_nominal_unit=m^3  liquid_mass_specify=off  liquid_mass_priority=None  liquid_mass=5 kg  liquid_mass_nominal_specify=off  liquid_mass_nominal_value=1  liquid_mass_nominal_unit=kg  p_I_specify=on  p_I_priority=High  p_I=5*0.101303 MPa  p_I_nominal_specify=off  p_I_nominal_value=1  p_I_nominal_unit=MPa  T_I_specify=on  T_I_priority=High  T_I="max(274,value(modelParam.WetBulbT,\"K\")) K"  T_I_nominal_specify=off  T_I_nominal_value=1  T_I_nominal_unit=K
      settings: InternalSimscapePortConfiguration="{\"Bottom\":[],\"Left\":[],\"Right\":[{\"id\":\"A\",\"label\":\"A\",\"type\":\"foundation.thermal_liquid.thermal_liquid\"},{\"id\":\"H\",\"label\":\"H\",\"type\":\"foundation.thermal.thermal\"}],\"Top\":[]}"
  Perfect Insulator1 : fl_lib/Thermal/Thermal Elements/Perfect Insulator  T_specify=off  T_priority=None  T=293.15 K  T_nominal_specify=off  T_nominal_value=1  T_nominal_unit=K
  " " : PMIOPort  Side=Left
  connections:
  Perfect Insulator1/LConn1 -- Expansion Tank/RConn2
  " "/RConn1 -- Expansion Tank/RConn1

== system DesignTemperatureControlForDataCenter/External Pump ==
  Ideal Angular Velocity Source : fl_lib/Mechanical/Mechanical Sources/Ideal Angular Velocity Source
  Ideal Torque Sensor : fl_lib/Mechanical/Mechanical Sensors/Ideal Torque Sensor
  Mechanical Rotational Reference : fl_lib/Mechanical/Rotational Elements/Mechanical Rotational Reference
  PS Product : fl_lib/Physical Signals/Functions/PS Product
  PS-Simulink Converter4 : nesl_utility/PS-Simulink Converter  PhysicalDomain=network_engine_domain  SubClassName=ps_output  LeftPortType=input  RightPortType=output  PseudoPeriodic=off  Frequencies=[]  VectorFormat=inherit  Unit=inherit  AffineConversion=off
  Pump Speed : fl_lib/Physical Signals/Functions/PS Gain  gain=2400 rpm
  C : PMIOPort  Side=Left
  R : PMIOPort  Port=2  Side=Left
  cmd : PMIOPort  Port=3  Side=Right
  P : Outport
  wires:
  PS-Simulink Converter4/1 -> P/1
  connections:
  C/RConn1 -- Ideal Angular Velocity Source/RConn2 -- Mechanical Rotational Reference/LConn1
  Pump Speed/RConn1 -- PS Product/LConn2 -- Ideal Angular Velocity Source/RConn1
  cmd/RConn1 -- Pump Speed/LConn1
  Ideal Angular Velocity Source/LConn1 -- Ideal Torque Sensor/LConn1
  Ideal Torque Sensor/RConn1 -- R/RConn1
  Ideal Torque Sensor/RConn2 -- PS Product/LConn1
  PS-Simulink Converter4/LConn1 -- PS Product/RConn1
